simulink model "magball2018"  (R2018a)
settings: Solver=VariableStepAuto  StartTime=0.0  StopTime=10.0  RelTol=1e-3
settings Model: Creator=vishn  LastModifiedBy=vishn
settings DataIOCC: ReturnWorkspaceOutputs=on
settings DebuggingCC: SFMachineParentedDataDiag=error
settings SFSimCC: SimUseLocalCustomCode=on
settings RTWCC: RTWUseLocalCustomCode=on

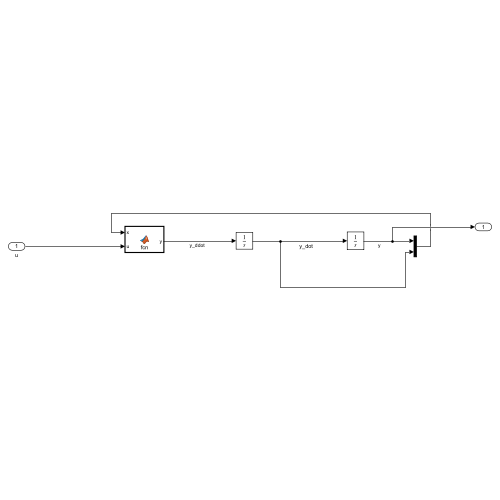
[thumbnail: Simulink's stored preview of the top-level diagram]
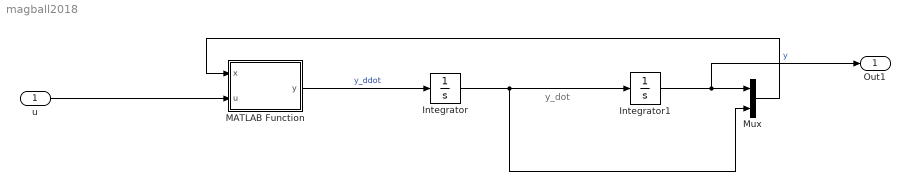
== system magball2018 ==
  note: y_dot
  u : Inport
  Integrator : Integrator
  Integrator1 : Integrator
  MATLAB Function : MATLAB Function  TreatAsAtomicUnit=on
  Mux : Mux  Inputs=2
  Out1 : Outport
  wires:
  u/1 -> MATLAB Function/2(u)
  MATLAB Function/1(y) -> Integrator/1  "y_ddot"
  Integrator/1 -> Mux/2, Integrator1/1
  Integrator1/1 -> Out1/1, Mux/1  "y"
  Mux/1 -> MATLAB Function/1(x)

== matlab function magball2018/MATLAB Function ==
  data: x input; u input; y output
function y = fcn(x, u)

y = 9.8 - ((u^2)/(x(1)^2));
